simulink model "untitled"  (R2022b)
settings: Solver=FixedStepAuto  StartTime=0.0  StopTime=0.3  FixedStep=1e-7  RelTol=1e-3
undefined symbols (not defined in the file): Ts
libraries: spsMosfetLib x12, simulink x11, spsControlledVoltageSourceLib x1, spsDCVoltageSourceLib x1, spsGroundLib x1, spsPermanentMagnetSynchronousMachineLib x1, spsSVPWMGenerator2LevelLib x1, spsdq0toAlphaBetaZeroLib x1, spspowerguiLib x1
(part 1 of 2)
settings Model: Creator=Javnson  LastModifiedBy=Javnson

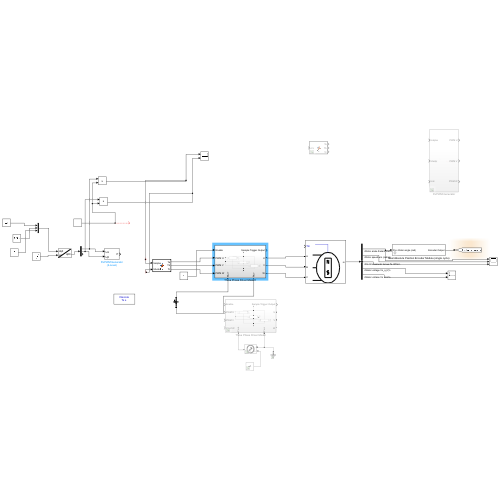
[thumbnail: Simulink's stored preview of the top-level diagram]
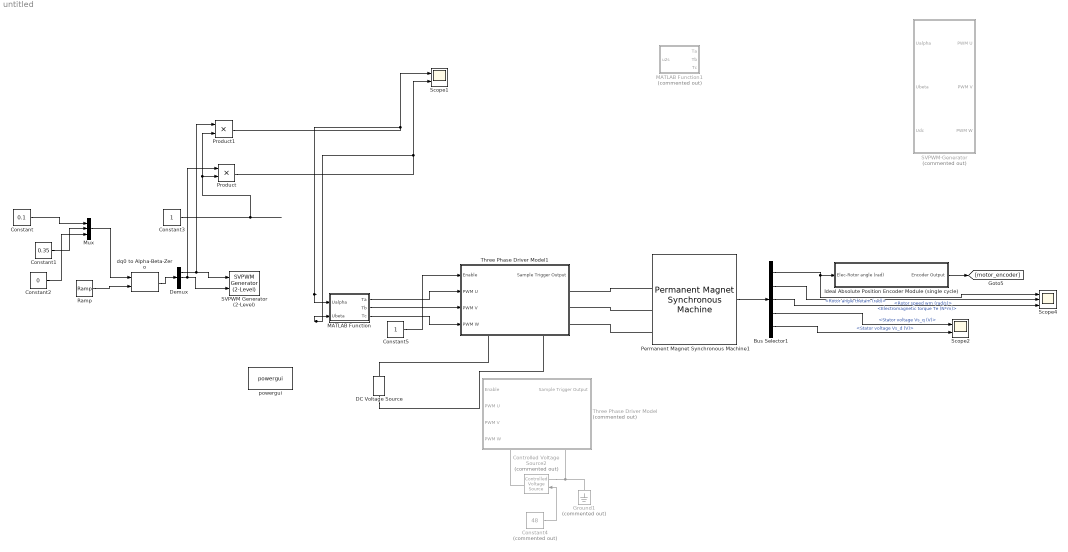
== system untitled ==
  Bus Selector1 : BusSelector  OutputSignals=Rotor angle thetam (rad),Rotor speed wm (rad/s),Electromagnetic torque Te (N*m),Stator voltage Vs_q (V),Stator voltage Vs_d (V)
  Constant : Constant  Value=0.1
  Constant1 : Constant  Value=0.35
  Constant2 : Constant  Value=0
  Constant3 : Constant
  Constant4 : Constant  Commented=on  Value=48
  Constant5 : Constant
  Controlled Voltage Source2 : spsControlledVoltageSourceLib/Controlled Voltage Source  Commented=on  Initialize=on  Source_Type=AC  Amplitude=0  Phase=0  Frequency=0  Measurements=None
  DC Voltage Source : spsDCVoltageSourceLib/DC Voltage Source  Amplitude=48  Measurements=None
  Demux : Demux  Outputs=3
  Ground1 : spsGroundLib/Ground  Commented=on  LConnTagsString=a
  Ideal Absolute Position Encoder Module (single cycle) : Subsystem  mask{ENCODER_BIT=17}
      mask DialogControl DescGroupVar Prompt: Ideal Absolute Position Encoder Module (single cycle)
      mask DialogControl DescTextVar Prompt: Avsolute Encoder transfer a motor mechanical angle (thetam, rad) to Absolute Encoder result. Generally, an absolute encoder has 17-bits or 23-bits resolution results.
      mask DialogControl ParameterGroupVar Prompt: 参数
      mask DialogControl Control2 Prompt: Absolute Encoder Resolution (bits):
  MATLAB Function : MATLAB Function  TreatAsAtomicUnit=on
  MATLAB Function1 : MATLAB Function  Commented=on  TreatAsAtomicUnit=on
  Mux : Mux  Inputs=3
  Permanent Magnet Synchronous Machine1 : spsPermanentMagnetSynchronousMachineLib/Permanent Magnet Synchronous Machine  NbPhases=3  FluxDistribution=Sinusoidal  RotorType=Round  MechanicalLoad=Torque Tm  PresetModel=No  ShowDetailedParameters=on  MeasurementBus=off  Resistance=0.18  Inductance=8.5e-3  dqInductances=[8.5e-3,8.5e-3]  La=0.000835  MachineConstant=Flux linkage established by magnets (V.s)  Flux=0.0714394  VoltageCst=51.8307  TorqueCst=0.42864  Flat=120  Mechanical=[0.000621417 0.000005 4 0]  PolePairs=4  InitialConditions=[0, 0, 0, 0]  InitialConditions5ph=[0 0 0 0 0 0]  RefAngle=Aligned with phase A axis (original Park)  IterativeDiscreteModel=Trapezoidal non iterative  TsBlock=-1  TsPowergui=0
  Product : Product
  Product1 : Product
  Ramp : simulink/Sources/Ramp  slope=40*pi  start=0  InitialOutput=0
  SVPWM Generator (2-Level) : spsSVPWMGenerator2LevelLib/SVPWM Generator (2-Level)  InputType=alpha-beta components  SwitchingPattern=Pattern #2  Fc=10e3  ParUref=[0.8 -30 50]  Ts=0
  SVPWM-Generator : Subsystem  Commented=on
  Scope1 : Scope  NumInputPorts=2
  Scope2 : Scope  NumInputPorts=2
  Scope4 : Scope  NumInputPorts=3
  Three Phase Driver Model : Subsystem  Commented=on
      settings: PortSchema="{\"entries\":[{\"content\":{\"sides\":[{\"content\":{\"connectorIds\":[\"In1\",\"In2\",\"In3\",\"In4\"]},\"type\":\"ConnectorPlacement.EquallySpacedRectSide\",\"uuid\":\"3ffcf095-7a60-4897-81b4-d3692ae6e2ab\"},{\"content\":{\"connectorIds\":[\"Out1\",\"RConn1\",\"RConn2\",\"RConn3\"],\"side\":\"RIGHT\"},\"type\":\"ConnectorPlacement.EquallySpacedRectSide\",\"uuid\":\"6e5cf4cf-b1b9-48ac-a692-0a8874277a23\"},{\"content\":{\"connectorIds\":[],\"side\":\"TOP\"},\"type\":\"ConnectorPlacement.EquallySpacedRectSide\",\"uuid\":\"9aa765f5-1b2f-406c-a04a-fab38ac2c4f7\"},{\"content\":{\"connectorIds\":[\"RConn4\",\"RConn5\"],\"side\":\"BOTTOM\"},\"type\":\"ConnectorPlacement.EquallySpacedRectSide\",\"uuid\":\"ff3856e6-d154-4ba2-8db0-f3c94a45cad8\"}]},\"type\":\"ConnectorPlacement.EquallySpacedConnector\",\"uuid\":\"490a993e-7d06-4faf-ab4a-bafd9b6172f2\"}],\"packageUris\":[\"http://schema.mathworks.com/mf0/Connector/R2020b\"],\"version\":\"1.0\"}"
  Three Phase Driver Model1 : Subsystem
      settings: PortSchema="{\"entries\":[{\"content\":{\"sides\":[{\"content\":{\"connectorIds\":[\"In1\",\"In2\",\"In3\",\"In4\"]},\"type\":\"ConnectorPlacement.EquallySpacedRectSide\",\"uuid\":\"3ffcf095-7a60-4897-81b4-d3692ae6e2ab\"},{\"content\":{\"connectorIds\":[\"Out1\",\"RConn1\",\"RConn2\",\"RConn3\"],\"side\":\"RIGHT\"},\"type\":\"ConnectorPlacement.EquallySpacedRectSide\",\"uuid\":\"6e5cf4cf-b1b9-48ac-a692-0a8874277a23\"},{\"content\":{\"connectorIds\":[],\"side\":\"TOP\"},\"type\":\"ConnectorPlacement.EquallySpacedRectSide\",\"uuid\":\"9aa765f5-1b2f-406c-a04a-fab38ac2c4f7\"},{\"content\":{\"connectorIds\":[\"RConn4\",\"RConn5\"],\"side\":\"BOTTOM\"},\"type\":\"ConnectorPlacement.EquallySpacedRectSide\",\"uuid\":\"ff3856e6-d154-4ba2-8db0-f3c94a45cad8\"}]},\"type\":\"ConnectorPlacement.EquallySpacedConnector\",\"uuid\":\"490a993e-7d06-4faf-ab4a-bafd9b6172f2\"}],\"packageUris\":[\"http://schema.mathworks.com/mf0/Connector/R2020b\"],\"version\":\"1.0\"}"
  dq0 to Alpha-Beta-Zero : spsdq0toAlphaBetaZeroLib/dq0 to Alpha-Beta-Zero  Alignment=Aligned with phase A axis
  powergui : spspowerguiLib/powergui  Priority=1  SimulationMode=Discrete  SampleTime=Ts  frequency=60  Iterations=50  frequencyindice=0  Pbase=100e6  ErrMax=1e-4  UnitsV=kV  UnitsW=MW  buscounter=0  FunctionMessages=off  echomessages=off  EnableUseOfTLC=off  CurrentSourceSwitches=off  DisableSnubberDevices=off  DisableRonSwitches=off  DisableVfSwitches=off  DisplayEquations=off  AutomaticDiscreteSolvers=off  SolverType=Tustin/Backward Euler (TBE)  Interpol=off  ExternalGateDelay=off  methode=off  Ts=100  x0status=blocks  SPID=on  SwTol=0  HookPort=off  NonlinearTolerance=1e-4  nMaxIteration=100  ContinueOnMaxIteration=off  RestoreLinks=warning  ResistiveCurrentMeasurement=off  Frange=[0:2:500]  Ylog=off  Xlog=on  ShowGrid=off  save=off  variable=ZData  structure=0  ZoomFFT=off  StartTime=0.0  cycles=1  DisplayStyle=1  fundamental=60  FreqAxis=off  MaxFrequency=1000  frequencyindicesteady=1  RmsSteady=1  display=off
  wires:
  Demux/1 -> Product1/1, SVPWM Generator (2-Level)/1
  Demux/2 -> Product/1, SVPWM Generator (2-Level)/2
  dq0 to Alpha-Beta-Zero/1 -> Demux/1
  Ramp/1 -> dq0 to Alpha-Beta-Zero/2
  Mux/1 -> dq0 to Alpha-Beta-Zero/1
  Constant/1 -> Mux/1
  Constant1/1 -> Mux/2
  Constant2/1 -> Mux/3
  Bus Selector1/2 -> Scope4/2  "<Rotor speed wm (rad/s)>"
  Bus Selector1/4 -> Scope2/1  "<Stator voltage Vs_q (V)>"
  Bus Selector1/5 -> Scope2/2  "<Stator voltage Vs_d (V)>"
  Ideal Absolute Position Encoder Module (single cycle)/1(Encoder Output) -> [motor_encoder]
  Permanent Magnet Synchronous Machine1/1 -> Bus Selector1/1
  Bus Selector1/1 -> Scope4/1, Ideal Absolute Position Encoder Module (single cycle)/1(Elec-Rotor angle (rad))  "<Rotor angle thetam (rad)>"
  Bus Selector1/3 -> Scope4/3  "<Electromagnetic torque Te (N*m)>"
  Constant4/1 -> Controlled Voltage Source2/1
  Product/1 -> MATLAB Function/2(Ubeta), Scope1/2
  Constant3/1 -> Product/2, Product1/2
  MATLAB Function/1(Ta) -> Three Phase Driver Model1/2(PWM U)
  MATLAB Function/2(Tb) -> Three Phase Driver Model1/3(PWM V)
  MATLAB Function/3(Tc) -> Three Phase Driver Model1/4(PWM W)
  Constant5/1 -> Three Phase Driver Model1/1(Enable)
  Product1/1 -> Scope1/1, MATLAB Function/1(Ualpha)
  connections:
  Permanent Magnet Synchronous Machine1/LConn1 -- Three Phase Driver Model1/RConn1
  Permanent Magnet Synchronous Machine1/LConn2 -- Three Phase Driver Model1/RConn2
  Permanent Magnet Synchronous Machine1/LConn3 -- Three Phase Driver Model1/RConn3
  DC Voltage Source/RConn1 -- Three Phase Driver Model1/RConn4
  DC Voltage Source/LConn1 -- Three Phase Driver Model1/RConn5
  Ground1/LConn1 -- Controlled Voltage Source2/LConn1 -- Three Phase Driver Model/RConn5
  Controlled Voltage Source2/RConn1 -- Three Phase Driver Model/RConn4

== system untitled/Ideal Absolute Position Encoder Module (single cycle) ==
  Elec-Rotor angle (rad) : Inport
  Data Type Conversion : DataTypeConversion  OutDataTypeStr=uint32  SaturateOnIntegerOverflow=off  RndMeth=Floor
  Gain : Gain  Gain=1/2/pi
  Type Conversion : Gain  Gain=2^ENCODER_BIT
  Encoder Output : Outport
  wires:
  Gain/1 -> Type Conversion/1
  Type Conversion/1 -> Data Type Conversion/1
  Data Type Conversion/1 -> Encoder Output/1
  Elec-Rotor angle (rad)/1 -> Gain/1

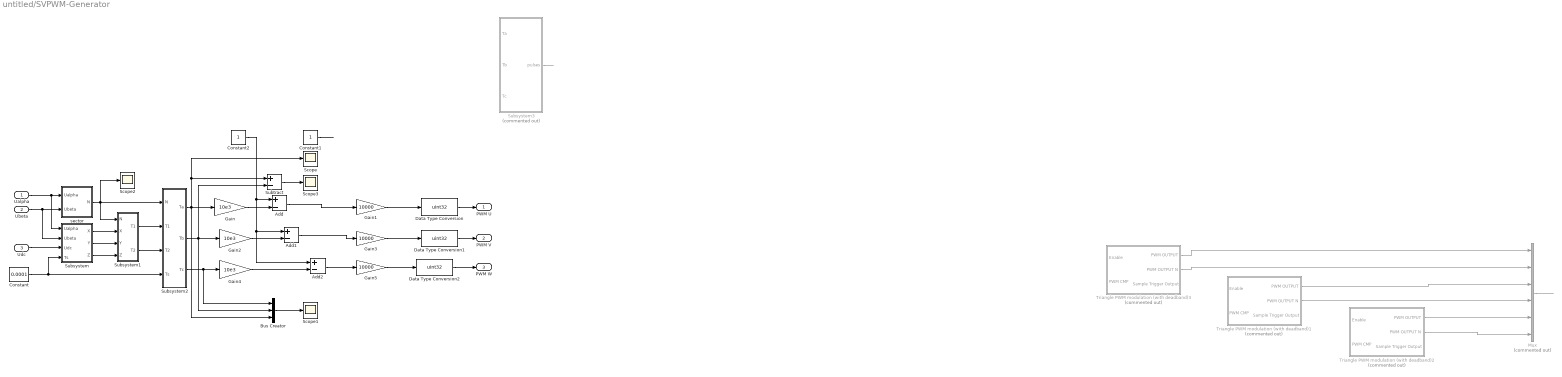
== system untitled/SVPWM-Generator ==
  Ualpha : Inport
  Ubeta : Inport  Port=2
  Udc : Inport  Port=3
  Add : Sum  Inputs=+-
  Add1 : Sum  Inputs=+-
  Add2 : Sum  Inputs=+-
  Bus Creator : BusCreator  Inputs=3
  Constant : Constant  Value=0.0001
  Constant1 : Constant
  Constant2 : Constant
  Data Type Conversion : DataTypeConversion  OutDataTypeStr=uint32  SaturateOnIntegerOverflow=off  RndMeth=Floor
  Data Type Conversion1 : DataTypeConversion  OutDataTypeStr=uint32  SaturateOnIntegerOverflow=off  RndMeth=Floor
  Data Type Conversion2 : DataTypeConversion  OutDataTypeStr=uint32  SaturateOnIntegerOverflow=off  RndMeth=Floor
  Gain : Gain  Gain=10e3
  Gain1 : Gain  Gain=10000
  Gain2 : Gain  Gain=10e3
  Gain3 : Gain  Gain=10000
  Gain4 : Gain  Gain=10e3
  Gain5 : Gain  Gain=10000
  Mux : Mux  Commented=on  Inputs=6
  Scope{,1..3} (4 alike) : Scope
  Subsystem : Subsystem
  Subsystem1 : Subsystem
  Subsystem2 : Subsystem
  Subsystem3 : Subsystem  Commented=on
  Subtract : Sum  Inputs=+-
  Triangle PWM modulation (with deadband)1 : Subsystem  Commented=on  mask{fswitch=10e3, CMP_MAX=10000, Deadband_Upper=0, Deadband_Lower=0, Parameter4=0}
      mask prompts: Parameter4 "Deadband Time: (μs)"
      mask Callback Deadband_Upper: %dead_cmp_param = get_param('DEADBAND_CMP','Value');
      mask DialogControl DescGroupVar Prompt: PWM Modulator
      mask DialogControl DescTextVar Prompt: PWM Modulator. Input PWM compare register value, output ADC trigger signal, PWM output and negtive PWM output.
      mask DialogControl ParameterGroupVar Prompt: 参数
      mask DialogControl Control2 Prompt: PWM Frequency (Hz) :
      mask DialogControl Control4 Prompt: Full Scale PWM Compare value:
      mask DialogControl Control5 Prompt: (whole period is 2 * CMP_MAX ticks)
      mask DialogControl Control3 Prompt: Deadband Range Set (CMP Value):
      mask DialogControl Control6 Prompt: Single side deadband time: DEADBAND_CMP/2/CMP_MAX/fswitch
  Triangle PWM modulation (with deadband)2 : Subsystem  Commented=on  mask{fswitch=10e3, CMP_MAX=10000, Deadband_Upper=0, Deadband_Lower=0, Parameter4=0}
      mask prompts: Parameter4 "Deadband Time: (μs)"
      mask Callback Deadband_Upper: %dead_cmp_param = get_param('DEADBAND_CMP','Value');
      mask DialogControl DescGroupVar Prompt: PWM Modulator
      mask DialogControl DescTextVar Prompt: PWM Modulator. Input PWM compare register value, output ADC trigger signal, PWM output and negtive PWM output.
      mask DialogControl ParameterGroupVar Prompt: 参数
      mask DialogControl Control2 Prompt: PWM Frequency (Hz) :
      mask DialogControl Control4 Prompt: Full Scale PWM Compare value:
      mask DialogControl Control5 Prompt: (whole period is 2 * CMP_MAX ticks)
      mask DialogControl Control3 Prompt: Deadband Range Set (CMP Value):
      mask DialogControl Control6 Prompt: Single side deadband time: DEADBAND_CMP/2/CMP_MAX/fswitch
  Triangle PWM modulation (with deadband)3 : Subsystem  Commented=on  mask{fswitch=10e3, CMP_MAX=10000, Deadband_Upper=0, Deadband_Lower=0, Parameter4=0}
      mask prompts: Parameter4 "Deadband Time: (μs)"
      mask Callback Deadband_Upper: %dead_cmp_param = get_param('DEADBAND_CMP','Value');
      mask DialogControl DescGroupVar Prompt: PWM Modulator
      mask DialogControl DescTextVar Prompt: PWM Modulator. Input PWM compare register value, output ADC trigger signal, PWM output and negtive PWM output.
      mask DialogControl ParameterGroupVar Prompt: 参数
      mask DialogControl Control2 Prompt: PWM Frequency (Hz) :
      mask DialogControl Control4 Prompt: Full Scale PWM Compare value:
      mask DialogControl Control5 Prompt: (whole period is 2 * CMP_MAX ticks)
      mask DialogControl Control3 Prompt: Deadband Range Set (CMP Value):
      mask DialogControl Control6 Prompt: Single side deadband time: DEADBAND_CMP/2/CMP_MAX/fswitch
  sector : Subsystem
  PWM U : Outport
  PWM V : Outport  Port=2
  PWM W : Outport  Port=3
  wires:
  sector/1(N) -> Scope2/1, Subsystem2/1(N), Subsystem1/1(N)
  Subsystem2/3(Tc) -> Gain4/1, Bus Creator/1
  Subsystem1/1(T1) -> Subsystem2/2(T1)
  Subsystem1/2(T2) -> Subsystem2/3(T2)
  Subsystem/1(X) -> Subsystem1/2(X)
  Subsystem3/1(pulses) -> ?
  Ubeta/1 -> Subsystem/2(Ubeta), sector/2(Ubeta)
  Constant/1 -> Subsystem2/4(Ts), Subsystem/4(Ts)
  Subsystem/2(Y) -> Subsystem1/3(Y)
  Subsystem/3(Z) -> Subsystem1/4(Z)
  Ualpha/1 -> Subsystem/1(Ualpha), sector/1(Ualpha)
  Subsystem2/1(Ta) -> Gain/1, Bus Creator/3, Subtract/1, Scope/1
  Udc/1 -> Subsystem/3(Udc)
  Bus Creator/1 -> Scope1/1
  Subtract/1 -> Scope3/1
  Gain1/1 -> Data Type Conversion/1
  Gain5/1 -> Data Type Conversion2/1
  Gain3/1 -> Data Type Conversion1/1
  Subsystem2/2(Tb) -> Gain2/1, Subtract/2, Bus Creator/2
  Constant1/1 -> ?
  Add/1 -> Gain1/1
  Gain/1 -> Add/2
  Add1/1 -> Gain3/1
  Gain2/1 -> Add1/2
  Add2/1 -> Gain5/1
  Gain4/1 -> Add2/2
  Constant2/1 -> Add2/1, Add1/1, Add/1
  Triangle PWM modulation (with deadband)2/2(PWM OUTPUT N) -> Mux/6
  ? -> Triangle PWM modulation (with deadband)1/1(Enable), Triangle PWM modulation (with deadband)2/1(Enable)
  ? -> Triangle PWM modulation (with deadband)3/1(Enable)
  Triangle PWM modulation (with deadband)1/1(PWM OUTPUT) -> Mux/3
  Mux/1 -> ?
  Triangle PWM modulation (with deadband)2/1(PWM OUTPUT) -> Mux/5
  Triangle PWM modulation (with deadband)3/2(PWM OUTPUT N) -> Mux/2
  ? -> Triangle PWM modulation (with deadband)1/2(PWM CMP)
  Triangle PWM modulation (with deadband)1/2(PWM OUTPUT N) -> Mux/4
  ? -> Triangle PWM modulation (with deadband)2/2(PWM CMP)
  Triangle PWM modulation (with deadband)3/1(PWM OUTPUT) -> Mux/1
  ? -> Triangle PWM modulation (with deadband)3/2(PWM CMP)
  Data Type Conversion/1 -> PWM U/1
  Data Type Conversion1/1 -> PWM V/1
  Data Type Conversion2/1 -> PWM W/1

== system untitled/Three Phase Driver Model ==
  Enable : Inport
  PWM U : Inport  Port=2
  PWM V : Inport  Port=3
  PWM W : Inport  Port=4
  Single Phase Full Bridge : Subsystem
      settings: PortSchema="{\"entries\":[{\"content\":{\"sides\":[{\"content\":{\"connectorIds\":[\"In1\",\"In2\"]},\"type\":\"ConnectorPlacement.EquallySpacedRectSide\",\"uuid\":\"20beeabc-b0ca-4337-b227-c7f02abd15d8\"},{\"content\":{\"connectorIds\":[\"Out1\",\"RConn1\"],\"side\":\"RIGHT\"},\"type\":\"ConnectorPlacement.EquallySpacedRectSide\",\"uuid\":\"a7923383-ac55-4621-ad1d-4d067c1fb84d\"},{\"content\":{\"connectorIds\":[\"LConn1\"],\"side\":\"TOP\"},\"type\":\"ConnectorPlacement.EquallySpacedRectSide\",\"uuid\":\"661bf0ae-1c96-4de8-96aa-28c06a0a56db\"},{\"content\":{\"connectorIds\":[\"RConn2\"],\"side\":\"BOTTOM\"},\"type\":\"ConnectorPlacement.EquallySpacedRectSide\",\"uuid\":\"fc2f6321-5787-4e1a-b5a2-65ed34db36b5\"}]},\"type\":\"ConnectorPlacement.EquallySpacedConnector\",\"uuid\":\"e2219b16-0a50-43ef-8183-c55a35d5a2a0\"}],\"packageUris\":[\"http://schema.mathworks.com/mf0/Connector/R2020b\"],\"version\":\"1.0\"}"
  Single Phase Full Bridge1 : Subsystem
      settings: PortSchema="{\"entries\":[{\"content\":{\"sides\":[{\"content\":{\"connectorIds\":[\"In1\",\"In2\"]},\"type\":\"ConnectorPlacement.EquallySpacedRectSide\",\"uuid\":\"20beeabc-b0ca-4337-b227-c7f02abd15d8\"},{\"content\":{\"connectorIds\":[\"Out1\",\"RConn1\"],\"side\":\"RIGHT\"},\"type\":\"ConnectorPlacement.EquallySpacedRectSide\",\"uuid\":\"a7923383-ac55-4621-ad1d-4d067c1fb84d\"},{\"content\":{\"connectorIds\":[\"LConn1\"],\"side\":\"TOP\"},\"type\":\"ConnectorPlacement.EquallySpacedRectSide\",\"uuid\":\"661bf0ae-1c96-4de8-96aa-28c06a0a56db\"},{\"content\":{\"connectorIds\":[\"RConn2\"],\"side\":\"BOTTOM\"},\"type\":\"ConnectorPlacement.EquallySpacedRectSide\",\"uuid\":\"fc2f6321-5787-4e1a-b5a2-65ed34db36b5\"}]},\"type\":\"ConnectorPlacement.EquallySpacedConnector\",\"uuid\":\"e2219b16-0a50-43ef-8183-c55a35d5a2a0\"}],\"packageUris\":[\"http://schema.mathworks.com/mf0/Connector/R2020b\"],\"version\":\"1.0\"}"
  Single Phase Full Bridge2 : Subsystem
      settings: PortSchema="{\"entries\":[{\"content\":{\"sides\":[{\"content\":{\"connectorIds\":[\"In1\",\"In2\"]},\"type\":\"ConnectorPlacement.EquallySpacedRectSide\",\"uuid\":\"20beeabc-b0ca-4337-b227-c7f02abd15d8\"},{\"content\":{\"connectorIds\":[\"Out1\",\"RConn1\"],\"side\":\"RIGHT\"},\"type\":\"ConnectorPlacement.EquallySpacedRectSide\",\"uuid\":\"a7923383-ac55-4621-ad1d-4d067c1fb84d\"},{\"content\":{\"connectorIds\":[\"LConn1\"],\"side\":\"TOP\"},\"type\":\"ConnectorPlacement.EquallySpacedRectSide\",\"uuid\":\"661bf0ae-1c96-4de8-96aa-28c06a0a56db\"},{\"content\":{\"connectorIds\":[\"RConn2\"],\"side\":\"BOTTOM\"},\"type\":\"ConnectorPlacement.EquallySpacedRectSide\",\"uuid\":\"fc2f6321-5787-4e1a-b5a2-65ed34db36b5\"}]},\"type\":\"ConnectorPlacement.EquallySpacedConnector\",\"uuid\":\"e2219b16-0a50-43ef-8183-c55a35d5a2a0\"}],\"packageUris\":[\"http://schema.mathworks.com/mf0/Connector/R2020b\"],\"version\":\"1.0\"}"
  Terminator : Terminator
  Terminator1 : Terminator
  U : PMIOPort  Side=Right
  V : PMIOPort  Port=2  Side=Right
  W : PMIOPort  Port=3  Side=Right
  Pwr+ : PMIOPort  Port=4  Side=Right
  Pwr- : PMIOPort  Port=5  Side=Right
  Sample Trigger Output : Outport
  wires:
  PWM W/1 -> Single Phase Full Bridge2/2(PWM CMP)
  Single Phase Full Bridge2/1(Sample Trigger Output) -> Terminator1/1
  Enable/1 -> Single Phase Full Bridge/1(Enable), Single Phase Full Bridge1/1(Enable), Single Phase Full Bridge2/1(Enable)
  Single Phase Full Bridge1/1(Sample Trigger Output) -> Terminator/1
  Single Phase Full Bridge/1(Sample Trigger Output) -> Sample Trigger Output/1
  PWM U/1 -> Single Phase Full Bridge/2(PWM CMP)
  PWM V/1 -> Single Phase Full Bridge1/2(PWM CMP)
  connections:
  Single Phase Full Bridge2/LConn1 -- Pwr+/RConn1 -- Single Phase Full Bridge1/LConn1 -- Single Phase Full Bridge/LConn1
  Single Phase Full Bridge2/RConn2 -- Pwr-/RConn1 -- Single Phase Full Bridge/RConn2 -- Single Phase Full Bridge1/RConn2
  Single Phase Full Bridge1/RConn1 -- V/RConn1
  Single Phase Full Bridge2/RConn1 -- W/RConn1
  Single Phase Full Bridge/RConn1 -- U/RConn1

== system untitled/Three Phase Driver Model1 ==
  Enable : Inport
  PWM U : Inport  Port=2
  PWM V : Inport  Port=3
  PWM W : Inport  Port=4
  Single Phase Full Bridge : Subsystem
      settings: PortSchema="{\"entries\":[{\"content\":{\"sides\":[{\"content\":{\"connectorIds\":[\"In1\",\"In2\"]},\"type\":\"ConnectorPlacement.EquallySpacedRectSide\",\"uuid\":\"20beeabc-b0ca-4337-b227-c7f02abd15d8\"},{\"content\":{\"connectorIds\":[\"Out1\",\"RConn1\"],\"side\":\"RIGHT\"},\"type\":\"ConnectorPlacement.EquallySpacedRectSide\",\"uuid\":\"a7923383-ac55-4621-ad1d-4d067c1fb84d\"},{\"content\":{\"connectorIds\":[\"LConn1\"],\"side\":\"TOP\"},\"type\":\"ConnectorPlacement.EquallySpacedRectSide\",\"uuid\":\"661bf0ae-1c96-4de8-96aa-28c06a0a56db\"},{\"content\":{\"connectorIds\":[\"RConn2\"],\"side\":\"BOTTOM\"},\"type\":\"ConnectorPlacement.EquallySpacedRectSide\",\"uuid\":\"fc2f6321-5787-4e1a-b5a2-65ed34db36b5\"}]},\"type\":\"ConnectorPlacement.EquallySpacedConnector\",\"uuid\":\"e2219b16-0a50-43ef-8183-c55a35d5a2a0\"}],\"packageUris\":[\"http://schema.mathworks.com/mf0/Connector/R2020b\"],\"version\":\"1.0\"}"
  Single Phase Full Bridge1 : Subsystem
      settings: PortSchema="{\"entries\":[{\"content\":{\"sides\":[{\"content\":{\"connectorIds\":[\"In1\",\"In2\"]},\"type\":\"ConnectorPlacement.EquallySpacedRectSide\",\"uuid\":\"20beeabc-b0ca-4337-b227-c7f02abd15d8\"},{\"content\":{\"connectorIds\":[\"Out1\",\"RConn1\"],\"side\":\"RIGHT\"},\"type\":\"ConnectorPlacement.EquallySpacedRectSide\",\"uuid\":\"a7923383-ac55-4621-ad1d-4d067c1fb84d\"},{\"content\":{\"connectorIds\":[\"LConn1\"],\"side\":\"TOP\"},\"type\":\"ConnectorPlacement.EquallySpacedRectSide\",\"uuid\":\"661bf0ae-1c96-4de8-96aa-28c06a0a56db\"},{\"content\":{\"connectorIds\":[\"RConn2\"],\"side\":\"BOTTOM\"},\"type\":\"ConnectorPlacement.EquallySpacedRectSide\",\"uuid\":\"fc2f6321-5787-4e1a-b5a2-65ed34db36b5\"}]},\"type\":\"ConnectorPlacement.EquallySpacedConnector\",\"uuid\":\"e2219b16-0a50-43ef-8183-c55a35d5a2a0\"}],\"packageUris\":[\"http://schema.mathworks.com/mf0/Connector/R2020b\"],\"version\":\"1.0\"}"
  Single Phase Full Bridge2 : Subsystem
      settings: PortSchema="{\"entries\":[{\"content\":{\"sides\":[{\"content\":{\"connectorIds\":[\"In1\",\"In2\"]},\"type\":\"ConnectorPlacement.EquallySpacedRectSide\",\"uuid\":\"20beeabc-b0ca-4337-b227-c7f02abd15d8\"},{\"content\":{\"connectorIds\":[\"Out1\",\"RConn1\"],\"side\":\"RIGHT\"},\"type\":\"ConnectorPlacement.EquallySpacedRectSide\",\"uuid\":\"a7923383-ac55-4621-ad1d-4d067c1fb84d\"},{\"content\":{\"connectorIds\":[\"LConn1\"],\"side\":\"TOP\"},\"type\":\"ConnectorPlacement.EquallySpacedRectSide\",\"uuid\":\"661bf0ae-1c96-4de8-96aa-28c06a0a56db\"},{\"content\":{\"connectorIds\":[\"RConn2\"],\"side\":\"BOTTOM\"},\"type\":\"ConnectorPlacement.EquallySpacedRectSide\",\"uuid\":\"fc2f6321-5787-4e1a-b5a2-65ed34db36b5\"}]},\"type\":\"ConnectorPlacement.EquallySpacedConnector\",\"uuid\":\"e2219b16-0a50-43ef-8183-c55a35d5a2a0\"}],\"packageUris\":[\"http://schema.mathworks.com/mf0/Connector/R2020b\"],\"version\":\"1.0\"}"
  Terminator : Terminator
  Terminator1 : Terminator
  U : PMIOPort  Side=Right
  V : PMIOPort  Port=2  Side=Right
  W : PMIOPort  Port=3  Side=Right
  Pwr+ : PMIOPort  Port=4  Side=Right
  Pwr- : PMIOPort  Port=5  Side=Right
  Sample Trigger Output : Outport
  wires:
  PWM W/1 -> Single Phase Full Bridge2/2(PWM CMP)
  Single Phase Full Bridge2/1(Sample Trigger Output) -> Terminator1/1
  Enable/1 -> Single Phase Full Bridge/1(Enable), Single Phase Full Bridge1/1(Enable), Single Phase Full Bridge2/1(Enable)
  Single Phase Full Bridge1/1(Sample Trigger Output) -> Terminator/1
  Single Phase Full Bridge/1(Sample Trigger Output) -> Sample Trigger Output/1
  PWM U/1 -> Single Phase Full Bridge/2(PWM CMP)
  PWM V/1 -> Single Phase Full Bridge1/2(PWM CMP)
  connections:
  Single Phase Full Bridge2/LConn1 -- Pwr+/RConn1 -- Single Phase Full Bridge1/LConn1 -- Single Phase Full Bridge/LConn1
  Single Phase Full Bridge2/RConn2 -- Pwr-/RConn1 -- Single Phase Full Bridge/RConn2 -- Single Phase Full Bridge1/RConn2
  Single Phase Full Bridge1/RConn1 -- V/RConn1
  Single Phase Full Bridge2/RConn1 -- W/RConn1
  Single Phase Full Bridge/RConn1 -- U/RConn1

== system untitled/SVPWM-Generator/Subsystem ==
  Ualpha : Inport
  Ubeta : Inport  Port=2
  Udc : Inport  Port=3
  Ts : Inport  Port=4
  Add : Sum
  Constant : Constant  Value=1.5
  Constant1 : Constant  Value=0.866
  Constant2 : Constant  Value=1.732
  Math Function : Math  Operator=reciprocal
  Product{,1..6} (7 alike) : Product
  Subtract : Sum  Inputs=+-
  X : Outport
  Y : Outport  Port=2
  Z : Outport  Port=3
  wires:
  Product1/1 -> Product4/2, Product5/2, Product6/2
  Ts/1 -> Product1/2
  Product6/1 -> Z/1
  Add/1 -> Product5/1
  Ualpha/1 -> Product/2
  Math Function/1 -> Product1/1
  Product2/1 -> Subtract/1, Add/2
  Product4/1 -> X/1
  Product3/1 -> Product4/1
  Constant/1 -> Product/1
  Constant1/1 -> Product2/1
  Ubeta/1 -> Product3/1, Product2/2
  Product5/1 -> Y/1
  Product/1 -> Add/1, Subtract/2
  Constant2/1 -> Product3/2
  Udc/1 -> Math Function/1
  Subtract/1 -> Product6/1

== system untitled/SVPWM-Generator/Subsystem1 ==
  N : Inport
  X : Inport  Port=2
  Y : Inport  Port=3
  Z : Inport  Port=4
  Gain : Gain  Gain=-1
  Gain1 : Gain  Gain=-1
  Gain2 : Gain  Gain=-1
  Multiport Switch : MultiPortSwitch  Inputs=6  SaturateOnIntegerOverflow=off  InputSameDT=off
  Multiport Switch1 : MultiPortSwitch  Inputs=6  SaturateOnIntegerOverflow=off  InputSameDT=off
  T1 : Outport
  T2 : Outport  Port=2
  wires:
  Multiport Switch1/1 -> T2/1
  X/1 -> Multiport Switch1/4, Multiport Switch/6, Gain/1
  Y/1 -> Gain1/1, Multiport Switch/3, Multiport Switch1/2
  Z/1 -> Gain2/1, Multiport Switch/2, Multiport Switch1/5
  Gain/1 -> Multiport Switch1/3, Multiport Switch/5
  Gain2/1 -> Multiport Switch/4, Multiport Switch1/7
  N/1 -> Multiport Switch1/1, Multiport Switch/1
  Gain1/1 -> Multiport Switch1/6, Multiport Switch/7
  Multiport Switch/1 -> T1/1

== system untitled/SVPWM-Generator/Subsystem2 ==
  N : Inport
  T1 : Inport  Port=2  Interpolate=off
  T2 : Inport  Port=3
  Ts : Inport  Port=4
  Add : Sum
  Add1 : Sum
  Constant : Constant  Value=0.25
  Constant1 : Constant  Value=0.5
  Constant2 : Constant  Value=0.5
  Multiport Switch : MultiPortSwitch  Inputs=6  SaturateOnIntegerOverflow=off  InputSameDT=off
  Multiport Switch1 : MultiPortSwitch  Inputs=6  SaturateOnIntegerOverflow=off  InputSameDT=off
  Multiport Switch2 : MultiPortSwitch  Inputs=6  SaturateOnIntegerOverflow=off  InputSameDT=off
  Product : Product
  Product1 : Product
  Product2 : Product
  Subtract : Sum  Inputs=--+
  Ta : Outport
  Tb : Outport  Port=2
  Tc : Outport  Port=3
  wires:
  Subtract/1 -> Product/1
  Product1/1 -> Add1/1
  T2/1 -> Product1/1, Subtract/2
  Product/1 -> Add/2, Multiport Switch2/5, Multiport Switch2/7, Multiport Switch/4, Multiport Switch/3, Multiport Switch1/2, Multiport Switch1/6
  Multiport Switch2/1 -> Tc/1
  Add1/1 -> Multiport Switch2/4, Multiport Switch2/2, Multiport Switch1/7, Multiport Switch1/3, Multiport Switch/6, Multiport Switch/5
  N/1 -> Multiport Switch2/1, Multiport Switch1/1, Multiport Switch/1
  Multiport Switch/1 -> Ta/1
  Constant/1 -> Product/2
  Constant2/1 -> Product2/2
  Add/1 -> Add1/2, Multiport Switch1/5, Multiport Switch/7, Multiport Switch/2, Multiport Switch1/4, Multiport Switch2/6, Multiport Switch2/3
  Multiport Switch1/1 -> Tb/1
  Product2/1 -> Add/1
  Constant1/1 -> Product1/2
  T1/1 -> Product2/1, Subtract/1
  Ts/1 -> Subtract/3

== system untitled/SVPWM-Generator/Subsystem3 ==
  Ta : Inport
  Tb : Inport  Port=2
  Tc : Inport  Port=3
  Bus Creator : BusCreator  Inputs=2
  Data Type Conversion : DataTypeConversion  OutDataTypeStr=boolean  SaturateOnIntegerOverflow=off  RndMeth=Floor  LockScale=on
  Data Type Conversion1 : DataTypeConversion  OutDataTypeStr=boolean  SaturateOnIntegerOverflow=off  RndMeth=Floor  LockScale=on
  Data Type Conversion2 : DataTypeConversion  OutDataTypeStr=boolean  SaturateOnIntegerOverflow=off  RndMeth=Floor  LockScale=on
  Logical Operator : Logic  Operator=NOT  AllPortsSameDT=off  OutDataTypeStr=boolean
  Logical Operator1 : Logic  Operator=NOT  AllPortsSameDT=off  OutDataTypeStr=boolean
  Logical Operator2 : Logic  Operator=NOT  AllPortsSameDT=off  OutDataTypeStr=boolean
  Mux : Mux  Inputs=6
  Relay : Relay
  Relay1 : Relay
  Relay2 : Relay
  Repeating Sequence : simulink/Sources/Repeating Sequence  rep_seq_t=[0 0.0001 0.0002]  rep_seq_y=[0 0.0001 0]
  Scope : Scope
  Subtract : Sum  Inputs=-+
  Subtract1 : Sum  Inputs=-+
  Subtract2 : Sum  Inputs=-+
  pulses : Outport
  wires:
  Data Type Conversion2/1 -> Mux/5
  Subtract1/1 -> Relay1/1
  Mux/1 -> pulses/1
  Data Type Conversion1/1 -> Mux/3
  Logical Operator2/1 -> Mux/6
  Relay/1 -> Logical Operator/1, Data Type Conversion/1
  Relay2/1 -> Logical Operator2/1, Data Type Conversion2/1
  Logical Operator/1 -> Bus Creator/2, Mux/2
  Relay1/1 -> Logical Operator1/1, Data Type Conversion1/1
  Repeating Sequence/1 -> Subtract/2, Subtract1/2, Subtract2/2
  Data Type Conversion/1 -> Bus Creator/1, Mux/1
  Logical Operator1/1 -> Mux/4
  Ta/1 -> Subtract/1
  Subtract2/1 -> Relay2/1
  Tb/1 -> Subtract1/1
  Subtract/1 -> Relay/1
  Tc/1 -> Subtract2/1
  Bus Creator/1 -> Scope/1

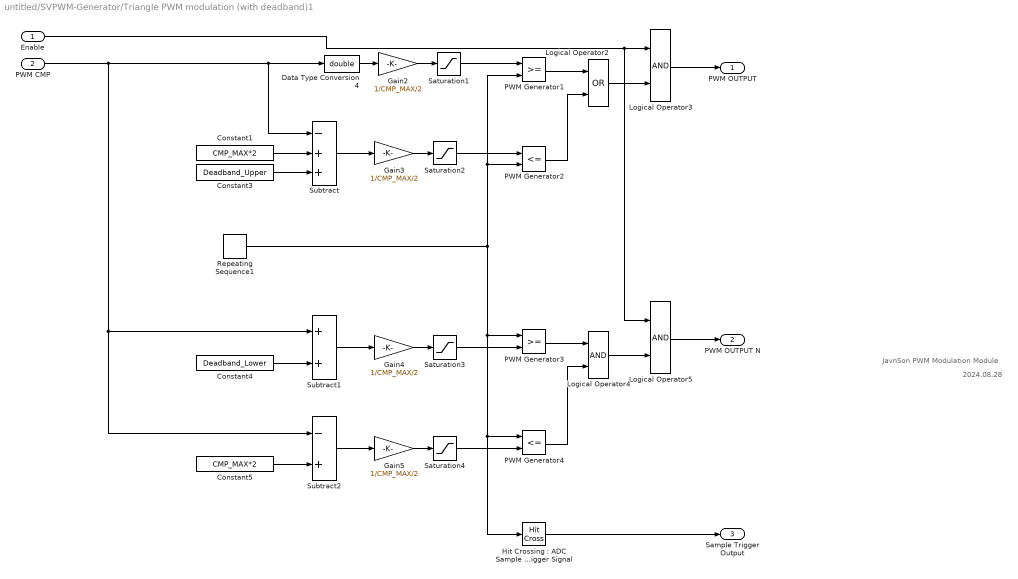
== system untitled/SVPWM-Generator/Triangle PWM modulation (with deadband)1 ==
  note: 2024.08.28
  note: JavnSon PWM Modulation Module
  Enable : Inport
  PWM CMP : Inport  Port=2
  Constant1 : Constant  Value=CMP_MAX*2
  Constant3 : Constant  Value=Deadband_Upper
  Constant4 : Constant  Value=Deadband_Lower
  Constant5 : Constant  Value=CMP_MAX*2
  Data Type Conversion4 : DataTypeConversion  OutDataTypeStr=double  SaturateOnIntegerOverflow=off  RndMeth=Floor
  Gain{2..5} (4 alike) : Gain  Gain=1/CMP_MAX/2
  Hit Crossing：ADC Sample Trigger Signal : HitCross  HitCrossingOffset=0.5  HitCrossingDirection=rising
  Logical Operator2 : Logic  Operator=OR  AllPortsSameDT=off  OutDataTypeStr=boolean
  Logical Operator3 : Logic  AllPortsSameDT=off  OutDataTypeStr=boolean
  Logical Operator4 : Logic  AllPortsSameDT=off  OutDataTypeStr=boolean
  Logical Operator5 : Logic  AllPortsSameDT=off  OutDataTypeStr=boolean
  PWM Generator1 : RelationalOperator  OutDataTypeStr=boolean  InputSameDT=off
  PWM Generator2 : RelationalOperator  Operator=<=  OutDataTypeStr=boolean  InputSameDT=off
  PWM Generator3 : RelationalOperator  OutDataTypeStr=boolean  InputSameDT=off
  PWM Generator4 : RelationalOperator  Operator=<=  OutDataTypeStr=boolean  InputSameDT=off
  Repeating Sequence1 : simulink/Sources/Repeating Sequence  rep_seq_t=[0, 1/2/fswitch, 1/fswitch ]  rep_seq_y=[0, 0.5, 1]
  Saturation{1..4} (4 alike) : Saturate  UpperLimit=1  LowerLimit=0
  Subtract : Sum  Inputs=-++
  Subtract1 : Sum
  Subtract2 : Sum  Inputs=-+
  PWM OUTPUT : Outport
  PWM OUTPUT N : Outport  Port=2
  Sample Trigger Output : Outport  Port=3
  wires:
  PWM CMP/1 -> Subtract2/1, Subtract1/1, Subtract/1, Data Type Conversion4/1
  Data Type Conversion4/1 -> Gain2/1
  Gain2/1 -> Saturation1/1
  Saturation1/1 -> PWM Generator1/1
  PWM Generator1/1 -> Logical Operator2/1
  Logical Operator2/1 -> Logical Operator3/2
  Constant1/1 -> Subtract/2
  Constant3/1 -> Subtract/3
  PWM Generator2/1 -> Logical Operator2/2
  Gain3/1 -> Saturation2/1
  Subtract/1 -> Gain3/1
  Saturation2/1 -> PWM Generator2/1
  Constant4/1 -> Subtract1/2
  Gain4/1 -> Saturation3/1
  Subtract1/1 -> Gain4/1
  Saturation3/1 -> PWM Generator3/2
  PWM Generator3/1 -> Logical Operator4/1
  Constant5/1 -> Subtract2/2
  Saturation4/1 -> PWM Generator4/2
  Gain5/1 -> Saturation4/1
  Subtract2/1 -> Gain5/1
  PWM Generator4/1 -> Logical Operator4/2
  Logical Operator4/1 -> Logical Operator5/2
  Repeating Sequence1/1 -> PWM Generator2/2, PWM Generator1/2, PWM Generator3/1, Hit Crossing：ADC Sample Trigger Signal/1, PWM Generator4/1
  Enable/1 -> Logical Operator5/1, Logical Operator3/1
  Logical Operator5/1 -> PWM OUTPUT N/1
  Logical Operator3/1 -> PWM OUTPUT/1
  Hit Crossing：ADC Sample Trigger Signal/1 -> Sample Trigger Output/1

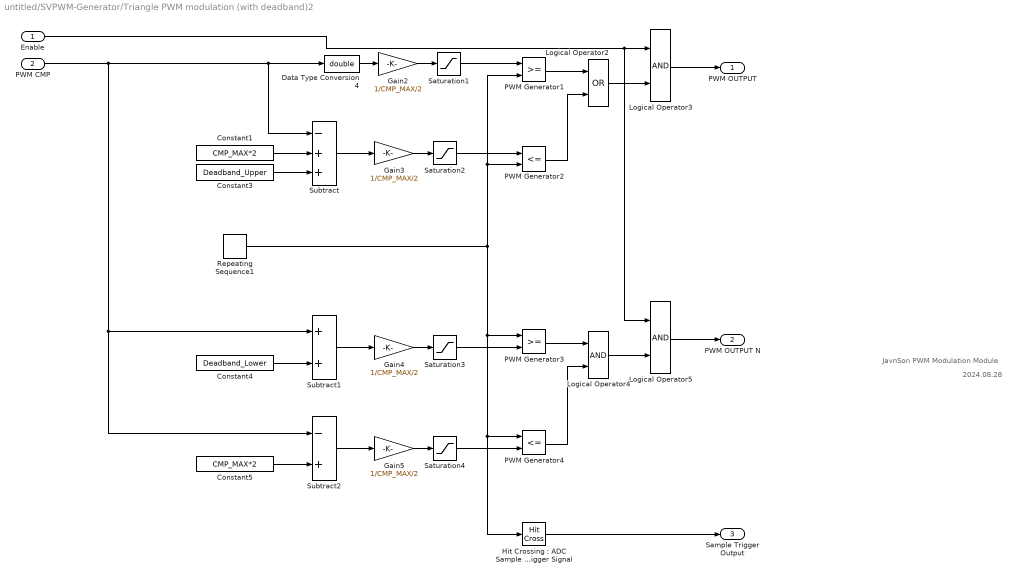
== system untitled/SVPWM-Generator/Triangle PWM modulation (with deadband)2 ==
  note: 2024.08.28
  note: JavnSon PWM Modulation Module
  Enable : Inport
  PWM CMP : Inport  Port=2
  Constant1 : Constant  Value=CMP_MAX*2
  Constant3 : Constant  Value=Deadband_Upper
  Constant4 : Constant  Value=Deadband_Lower
  Constant5 : Constant  Value=CMP_MAX*2
  Data Type Conversion4 : DataTypeConversion  OutDataTypeStr=double  SaturateOnIntegerOverflow=off  RndMeth=Floor
  Gain{2..5} (4 alike) : Gain  Gain=1/CMP_MAX/2
  Hit Crossing：ADC Sample Trigger Signal : HitCross  HitCrossingOffset=0.5  HitCrossingDirection=rising
  Logical Operator2 : Logic  Operator=OR  AllPortsSameDT=off  OutDataTypeStr=boolean
  Logical Operator3 : Logic  AllPortsSameDT=off  OutDataTypeStr=boolean
  Logical Operator4 : Logic  AllPortsSameDT=off  OutDataTypeStr=boolean
  Logical Operator5 : Logic  AllPortsSameDT=off  OutDataTypeStr=boolean
  PWM Generator1 : RelationalOperator  OutDataTypeStr=boolean  InputSameDT=off
  PWM Generator2 : RelationalOperator  Operator=<=  OutDataTypeStr=boolean  InputSameDT=off
  PWM Generator3 : RelationalOperator  OutDataTypeStr=boolean  InputSameDT=off
  PWM Generator4 : RelationalOperator  Operator=<=  OutDataTypeStr=boolean  InputSameDT=off
  Repeating Sequence1 : simulink/Sources/Repeating Sequence  rep_seq_t=[0, 1/2/fswitch, 1/fswitch ]  rep_seq_y=[0, 0.5, 1]
  Saturation{1..4} (4 alike) : Saturate  UpperLimit=1  LowerLimit=0
  Subtract : Sum  Inputs=-++
  Subtract1 : Sum
  Subtract2 : Sum  Inputs=-+
  PWM OUTPUT : Outport
  PWM OUTPUT N : Outport  Port=2
  Sample Trigger Output : Outport  Port=3
  wires:
  PWM CMP/1 -> Subtract2/1, Subtract1/1, Subtract/1, Data Type Conversion4/1
  Data Type Conversion4/1 -> Gain2/1
  Gain2/1 -> Saturation1/1
  Saturation1/1 -> PWM Generator1/1
  PWM Generator1/1 -> Logical Operator2/1
  Logical Operator2/1 -> Logical Operator3/2
  Constant1/1 -> Subtract/2
  Constant3/1 -> Subtract/3
  PWM Generator2/1 -> Logical Operator2/2
  Gain3/1 -> Saturation2/1
  Subtract/1 -> Gain3/1
  Saturation2/1 -> PWM Generator2/1
  Constant4/1 -> Subtract1/2
  Gain4/1 -> Saturation3/1
  Subtract1/1 -> Gain4/1
  Saturation3/1 -> PWM Generator3/2
  PWM Generator3/1 -> Logical Operator4/1
  Constant5/1 -> Subtract2/2
  Saturation4/1 -> PWM Generator4/2
  Gain5/1 -> Saturation4/1
  Subtract2/1 -> Gain5/1
  PWM Generator4/1 -> Logical Operator4/2
  Logical Operator4/1 -> Logical Operator5/2
  Repeating Sequence1/1 -> PWM Generator2/2, PWM Generator1/2, PWM Generator3/1, Hit Crossing：ADC Sample Trigger Signal/1, PWM Generator4/1
  Enable/1 -> Logical Operator5/1, Logical Operator3/1
  Logical Operator5/1 -> PWM OUTPUT N/1
  Logical Operator3/1 -> PWM OUTPUT/1
  Hit Crossing：ADC Sample Trigger Signal/1 -> Sample Trigger Output/1

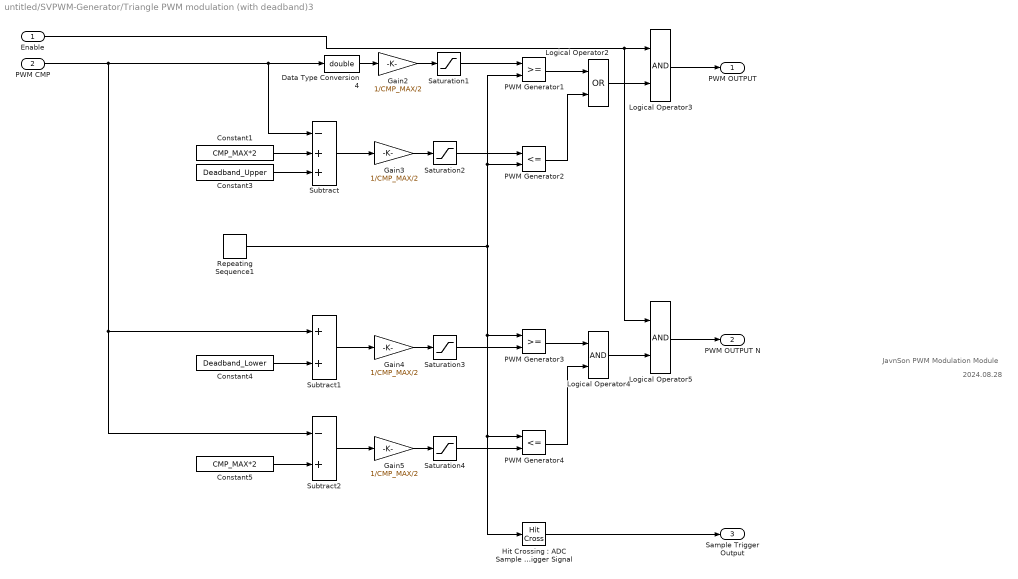
== system untitled/SVPWM-Generator/Triangle PWM modulation (with deadband)3 ==
  note: 2024.08.28
  note: JavnSon PWM Modulation Module
  Enable : Inport
  PWM CMP : Inport  Port=2
  Constant1 : Constant  Value=CMP_MAX*2
  Constant3 : Constant  Value=Deadband_Upper
  Constant4 : Constant  Value=Deadband_Lower
  Constant5 : Constant  Value=CMP_MAX*2
  Data Type Conversion4 : DataTypeConversion  OutDataTypeStr=double  SaturateOnIntegerOverflow=off  RndMeth=Floor
  Gain{2..5} (4 alike) : Gain  Gain=1/CMP_MAX/2
  Hit Crossing：ADC Sample Trigger Signal : HitCross  HitCrossingOffset=0.5  HitCrossingDirection=rising
  Logical Operator2 : Logic  Operator=OR  AllPortsSameDT=off  OutDataTypeStr=boolean
  Logical Operator3 : Logic  AllPortsSameDT=off  OutDataTypeStr=boolean
  Logical Operator4 : Logic  AllPortsSameDT=off  OutDataTypeStr=boolean
  Logical Operator5 : Logic  AllPortsSameDT=off  OutDataTypeStr=boolean
  PWM Generator1 : RelationalOperator  OutDataTypeStr=boolean  InputSameDT=off
  PWM Generator2 : RelationalOperator  Operator=<=  OutDataTypeStr=boolean  InputSameDT=off
  PWM Generator3 : RelationalOperator  OutDataTypeStr=boolean  InputSameDT=off
  PWM Generator4 : RelationalOperator  Operator=<=  OutDataTypeStr=boolean  InputSameDT=off
  Repeating Sequence1 : simulink/Sources/Repeating Sequence  rep_seq_t=[0, 1/2/fswitch, 1/fswitch ]  rep_seq_y=[0, 0.5, 1]
  Saturation{1..4} (4 alike) : Saturate  UpperLimit=1  LowerLimit=0
  Subtract : Sum  Inputs=-++
  Subtract1 : Sum
  Subtract2 : Sum  Inputs=-+
  PWM OUTPUT : Outport
  PWM OUTPUT N : Outport  Port=2
  Sample Trigger Output : Outport  Port=3
  wires:
  PWM CMP/1 -> Subtract2/1, Subtract1/1, Subtract/1, Data Type Conversion4/1
  Data Type Conversion4/1 -> Gain2/1
  Gain2/1 -> Saturation1/1
  Saturation1/1 -> PWM Generator1/1
  PWM Generator1/1 -> Logical Operator2/1
  Logical Operator2/1 -> Logical Operator3/2
  Constant1/1 -> Subtract/2
  Constant3/1 -> Subtract/3
  PWM Generator2/1 -> Logical Operator2/2
  Gain3/1 -> Saturation2/1
  Subtract/1 -> Gain3/1
  Saturation2/1 -> PWM Generator2/1
  Constant4/1 -> Subtract1/2
  Gain4/1 -> Saturation3/1
  Subtract1/1 -> Gain4/1
  Saturation3/1 -> PWM Generator3/2
  PWM Generator3/1 -> Logical Operator4/1
  Constant5/1 -> Subtract2/2
  Saturation4/1 -> PWM Generator4/2
  Gain5/1 -> Saturation4/1
  Subtract2/1 -> Gain5/1
  PWM Generator4/1 -> Logical Operator4/2
  Logical Operator4/1 -> Logical Operator5/2
  Repeating Sequence1/1 -> PWM Generator2/2, PWM Generator1/2, PWM Generator3/1, Hit Crossing：ADC Sample Trigger Signal/1, PWM Generator4/1
  Enable/1 -> Logical Operator5/1, Logical Operator3/1
  Logical Operator5/1 -> PWM OUTPUT N/1
  Logical Operator3/1 -> PWM OUTPUT/1
  Hit Crossing：ADC Sample Trigger Signal/1 -> Sample Trigger Output/1

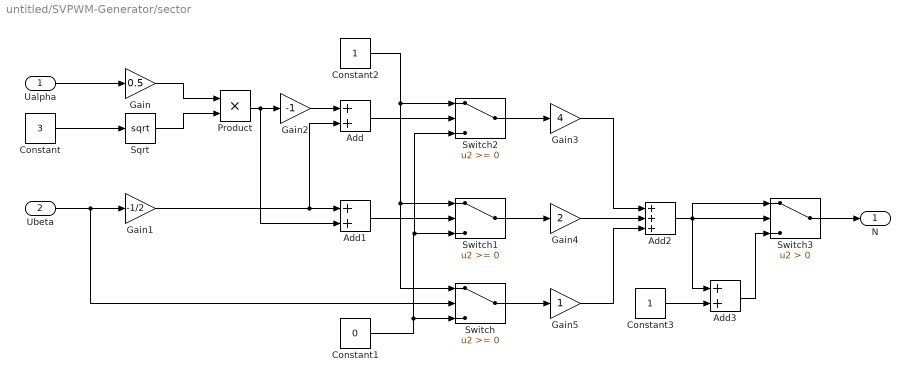
== system untitled/SVPWM-Generator/sector ==
  Ualpha : Inport
  Ubeta : Inport  Port=2
  Add : Sum
  Add1 : Sum
  Add2 : Sum  Inputs=+++
  Add3 : Sum
  Constant : Constant  Value=3
  Constant1 : Constant  Value=0
  Constant2 : Constant
  Constant3 : Constant
  Gain : Gain  Gain=0.5
  Gain1 : Gain  Gain=-1/2
  Gain2 : Gain  Gain=-1
  Gain3 : Gain  Gain=4
  Gain4 : Gain  Gain=2
  Gain5 : Gain
  Product : Product
  Sqrt : Sqrt
  Switch : Switch  SaturateOnIntegerOverflow=off  InputSameDT=off
  Switch1 : Switch  SaturateOnIntegerOverflow=off  InputSameDT=off
  Switch2 : Switch  SaturateOnIntegerOverflow=off  InputSameDT=off
  Switch3 : Switch  Criteria=u2 > Threshold  SaturateOnIntegerOverflow=off  InputSameDT=off
  N : Outport
  wires:
  Gain1/1 -> Add1/1, Add/2
  Constant1/1 -> Switch2/3, Switch1/3, Switch/3
  Gain2/1 -> Add/1
  Gain/1 -> Product/1
  Constant3/1 -> Add3/2
  Add/1 -> Switch2/2
  Product/1 -> Add1/2, Gain2/1
  Sqrt/1 -> Product/2
  Ubeta/1 -> Switch/2, Gain1/1
  Switch/1 -> Gain5/1
  Switch2/1 -> Gain3/1
  Add3/1 -> Switch3/3
  Add2/1 -> Switch3/1, Add3/1, Switch3/2
  Switch3/1 -> N/1
  Gain3/1 -> Add2/1
  Add1/1 -> Switch1/2
  Switch1/1 -> Gain4/1
  Gain4/1 -> Add2/2
  Constant/1 -> Sqrt/1
  Gain5/1 -> Add2/3
  Constant2/1 -> Switch/1, Switch1/1, Switch2/1
  Ualpha/1 -> Gain/1

== system untitled/Three Phase Driver Model/Single Phase Full Bridge ==
  Enable : Inport
  PWM CMP : Inport  Port=2
  Mosfet8 : spsMosfetLib/Mosfet  Ron=0.1  Lon=0  Rd=0.01  Vfd=0  IC=0  Rs=1e5  Cs=inf  Measurements=off
  Mosfet9 : spsMosfetLib/Mosfet  Ron=0.1  Lon=0  Rd=0.01  Vfd=0  IC=0  Rs=1e5  Cs=inf  Measurements=off
  Triangle PWM modulation (with deadband)3 : Subsystem  mask{fswitch=10e3, CMP_MAX=10000, Deadband_Upper=0, Deadband_Lower=0, Parameter4=0}
      mask prompts: Parameter4 "Deadband Time: (μs)"
      mask Callback Deadband_Upper: %dead_cmp_param = get_param('DEADBAND_CMP','Value');
      mask DialogControl DescGroupVar Prompt: PWM Modulator
      mask DialogControl DescTextVar Prompt: PWM Modulator. Input PWM compare register value, output ADC trigger signal, PWM output and negtive PWM output.
      mask DialogControl ParameterGroupVar Prompt: 参数
      mask DialogControl Control2 Prompt: PWM Frequency (Hz) :
      mask DialogControl Control4 Prompt: Full Scale PWM Compare value:
      mask DialogControl Control5 Prompt: (whole period is 2 * CMP_MAX ticks)
      mask DialogControl Control3 Prompt: Deadband Range Set (CMP Value):
      mask DialogControl Control6 Prompt: Single side deadband time: DEADBAND_CMP/2/CMP_MAX/fswitch
  D : PMIOPort  Side=Left
  Phase : PMIOPort  Port=2  Side=Right
  S : PMIOPort  Port=3  Side=Right
  Sample Trigger Output : Outport
  wires:
  Triangle PWM modulation (with deadband)3/1(PWM OUTPUT) -> Mosfet8/1
  Enable/1 -> Triangle PWM modulation (with deadband)3/1(Enable)
  Triangle PWM modulation (with deadband)3/3(Sample Trigger Output) -> Sample Trigger Output/1
  Triangle PWM modulation (with deadband)3/2(PWM OUTPUT N) -> Mosfet9/1
  PWM CMP/1 -> Triangle PWM modulation (with deadband)3/2(PWM CMP)
  connections:
  Mosfet8/LConn1 -- D/RConn1
  Mosfet9/LConn1 -- Phase/RConn1 -- Mosfet8/RConn1
  Mosfet9/RConn1 -- S/RConn1

== system untitled/Three Phase Driver Model/Single Phase Full Bridge1 ==
  Enable : Inport
  PWM CMP : Inport  Port=2
  Mosfet8 : spsMosfetLib/Mosfet  Ron=0.1  Lon=0  Rd=0.01  Vfd=0  IC=0  Rs=1e5  Cs=inf  Measurements=off
  Mosfet9 : spsMosfetLib/Mosfet  Ron=0.1  Lon=0  Rd=0.01  Vfd=0  IC=0  Rs=1e5  Cs=inf  Measurements=off
  Triangle PWM modulation (with deadband)3 : Subsystem  mask{fswitch=10e3, CMP_MAX=10000, Deadband_Upper=0, Deadband_Lower=0, Parameter4=0}
      mask prompts: Parameter4 "Deadband Time: (μs)"
      mask Callback Deadband_Upper: %dead_cmp_param = get_param('DEADBAND_CMP','Value');
      mask DialogControl DescGroupVar Prompt: PWM Modulator
      mask DialogControl DescTextVar Prompt: PWM Modulator. Input PWM compare register value, output ADC trigger signal, PWM output and negtive PWM output.
      mask DialogControl ParameterGroupVar Prompt: 参数
      mask DialogControl Control2 Prompt: PWM Frequency (Hz) :
      mask DialogControl Control4 Prompt: Full Scale PWM Compare value:
      mask DialogControl Control5 Prompt: (whole period is 2 * CMP_MAX ticks)
      mask DialogControl Control3 Prompt: Deadband Range Set (CMP Value):
      mask DialogControl Control6 Prompt: Single side deadband time: DEADBAND_CMP/2/CMP_MAX/fswitch
  D : PMIOPort  Side=Left
  Phase : PMIOPort  Port=2  Side=Right
  S : PMIOPort  Port=3  Side=Right
  Sample Trigger Output : Outport
  wires:
  Triangle PWM modulation (with deadband)3/1(PWM OUTPUT) -> Mosfet8/1
  Enable/1 -> Triangle PWM modulation (with deadband)3/1(Enable)
  Triangle PWM modulation (with deadband)3/3(Sample Trigger Output) -> Sample Trigger Output/1
  Triangle PWM modulation (with deadband)3/2(PWM OUTPUT N) -> Mosfet9/1
  PWM CMP/1 -> Triangle PWM modulation (with deadband)3/2(PWM CMP)
  connections:
  Mosfet8/LConn1 -- D/RConn1
  Mosfet8/RConn1 -- Mosfet9/LConn1 -- Phase/RConn1
  Mosfet9/RConn1 -- S/RConn1

== system untitled/Three Phase Driver Model/Single Phase Full Bridge2 ==
  Enable : Inport
  PWM CMP : Inport  Port=2
  Mosfet8 : spsMosfetLib/Mosfet  Ron=0.1  Lon=0  Rd=0.01  Vfd=0  IC=0  Rs=1e5  Cs=inf  Measurements=off
  Mosfet9 : spsMosfetLib/Mosfet  Ron=0.1  Lon=0  Rd=0.01  Vfd=0  IC=0  Rs=1e5  Cs=inf  Measurements=off
  Triangle PWM modulation (with deadband)3 : Subsystem  mask{fswitch=10e3, CMP_MAX=10000, Deadband_Upper=0, Deadband_Lower=0, Parameter4=0}
      mask prompts: Parameter4 "Deadband Time: (μs)"
      mask Callback Deadband_Upper: %dead_cmp_param = get_param('DEADBAND_CMP','Value');
      mask DialogControl DescGroupVar Prompt: PWM Modulator
      mask DialogControl DescTextVar Prompt: PWM Modulator. Input PWM compare register value, output ADC trigger signal, PWM output and negtive PWM output.
      mask DialogControl ParameterGroupVar Prompt: 参数
      mask DialogControl Control2 Prompt: PWM Frequency (Hz) :
      mask DialogControl Control4 Prompt: Full Scale PWM Compare value:
      mask DialogControl Control5 Prompt: (whole period is 2 * CMP_MAX ticks)
      mask DialogControl Control3 Prompt: Deadband Range Set (CMP Value):
      mask DialogControl Control6 Prompt: Single side deadband time: DEADBAND_CMP/2/CMP_MAX/fswitch
  D : PMIOPort  Side=Left
  Phase : PMIOPort  Port=2  Side=Right
  S : PMIOPort  Port=3  Side=Right
  Sample Trigger Output : Outport
  wires:
  Triangle PWM modulation (with deadband)3/1(PWM OUTPUT) -> Mosfet8/1
  Enable/1 -> Triangle PWM modulation (with deadband)3/1(Enable)
  Triangle PWM modulation (with deadband)3/3(Sample Trigger Output) -> Sample Trigger Output/1
  Triangle PWM modulation (with deadband)3/2(PWM OUTPUT N) -> Mosfet9/1
  PWM CMP/1 -> Triangle PWM modulation (with deadband)3/2(PWM CMP)
  connections:
  Mosfet8/LConn1 -- D/RConn1
  Mosfet8/RConn1 -- Mosfet9/LConn1 -- Phase/RConn1
  Mosfet9/RConn1 -- S/RConn1

== system untitled/Three Phase Driver Model1/Single Phase Full Bridge ==
  Enable : Inport
  PWM CMP : Inport  Port=2
  Mosfet8 : spsMosfetLib/Mosfet  Ron=1e-3  Lon=0  Rd=0.01  Vfd=0  IC=0  Rs=1e5  Cs=inf  Measurements=off
  Mosfet9 : spsMosfetLib/Mosfet  Ron=1e-3  Lon=0  Rd=0.01  Vfd=0  IC=0  Rs=1e5  Cs=inf  Measurements=off
  Triangle PWM modulation (with deadband)3 : Subsystem  mask{fswitch=10e3, CMP_MAX=10000, Deadband_Upper=0, Deadband_Lower=0, Parameter4=0}
      mask prompts: Parameter4 "Deadband Time: (μs)"
      mask Callback Deadband_Upper: %dead_cmp_param = get_param('DEADBAND_CMP','Value');
      mask DialogControl DescGroupVar Prompt: PWM Modulator
      mask DialogControl DescTextVar Prompt: PWM Modulator. Input PWM compare register value, output ADC trigger signal, PWM output and negtive PWM output.
      mask DialogControl ParameterGroupVar Prompt: 参数
      mask DialogControl Control2 Prompt: PWM Frequency (Hz) :
      mask DialogControl Control4 Prompt: Full Scale PWM Compare value:
      mask DialogControl Control5 Prompt: (whole period is 2 * CMP_MAX ticks)
      mask DialogControl Control3 Prompt: Deadband Range Set (CMP Value):
      mask DialogControl Control6 Prompt: Single side deadband time: DEADBAND_CMP/2/CMP_MAX/fswitch
  D : PMIOPort  Side=Left
  Phase : PMIOPort  Port=2  Side=Right
  S : PMIOPort  Port=3  Side=Right
  Sample Trigger Output : Outport
  wires:
  Triangle PWM modulation (with deadband)3/1(PWM OUTPUT) -> Mosfet8/1
  Enable/1 -> Triangle PWM modulation (with deadband)3/1(Enable)
  Triangle PWM modulation (with deadband)3/3(Sample Trigger Output) -> Sample Trigger Output/1
  Triangle PWM modulation (with deadband)3/2(PWM OUTPUT N) -> Mosfet9/1
  PWM CMP/1 -> Triangle PWM modulation (with deadband)3/2(PWM CMP)
  connections:
  Mosfet8/LConn1 -- D/RConn1
  Mosfet9/LConn1 -- Phase/RConn1 -- Mosfet8/RConn1
  Mosfet9/RConn1 -- S/RConn1

== system untitled/Three Phase Driver Model1/Single Phase Full Bridge1 ==
  Enable : Inport
  PWM CMP : Inport  Port=2
  Mosfet8 : spsMosfetLib/Mosfet  Ron=1e-3  Lon=0  Rd=0.01  Vfd=0  IC=0  Rs=1e5  Cs=inf  Measurements=off
  Mosfet9 : spsMosfetLib/Mosfet  Ron=1e-3  Lon=0  Rd=0.01  Vfd=0  IC=0  Rs=1e5  Cs=inf  Measurements=off
  Triangle PWM modulation (with deadband)3 : Subsystem  mask{fswitch=10e3, CMP_MAX=10000, Deadband_Upper=0, Deadband_Lower=0, Parameter4=0}
      mask prompts: Parameter4 "Deadband Time: (μs)"
      mask Callback Deadband_Upper: %dead_cmp_param = get_param('DEADBAND_CMP','Value');
      mask DialogControl DescGroupVar Prompt: PWM Modulator
      mask DialogControl DescTextVar Prompt: PWM Modulator. Input PWM compare register value, output ADC trigger signal, PWM output and negtive PWM output.
      mask DialogControl ParameterGroupVar Prompt: 参数
      mask DialogControl Control2 Prompt: PWM Frequency (Hz) :
      mask DialogControl Control4 Prompt: Full Scale PWM Compare value:
      mask DialogControl Control5 Prompt: (whole period is 2 * CMP_MAX ticks)
      mask DialogControl Control3 Prompt: Deadband Range Set (CMP Value):
      mask DialogControl Control6 Prompt: Single side deadband time: DEADBAND_CMP/2/CMP_MAX/fswitch
  D : PMIOPort  Side=Left
  Phase : PMIOPort  Port=2  Side=Right
  S : PMIOPort  Port=3  Side=Right
  Sample Trigger Output : Outport
  wires:
  Triangle PWM modulation (with deadband)3/1(PWM OUTPUT) -> Mosfet8/1
  Enable/1 -> Triangle PWM modulation (with deadband)3/1(Enable)
  Triangle PWM modulation (with deadband)3/3(Sample Trigger Output) -> Sample Trigger Output/1
  Triangle PWM modulation (with deadband)3/2(PWM OUTPUT N) -> Mosfet9/1
  PWM CMP/1 -> Triangle PWM modulation (with deadband)3/2(PWM CMP)
  connections:
  Mosfet8/LConn1 -- D/RConn1
  Mosfet8/RConn1 -- Mosfet9/LConn1 -- Phase/RConn1
  Mosfet9/RConn1 -- S/RConn1

== system untitled/Three Phase Driver Model1/Single Phase Full Bridge2 ==
  Enable : Inport
  PWM CMP : Inport  Port=2
  Mosfet8 : spsMosfetLib/Mosfet  Ron=1e-3  Lon=0  Rd=0.01  Vfd=0  IC=0  Rs=1e5  Cs=inf  Measurements=off
  Mosfet9 : spsMosfetLib/Mosfet  Ron=1e-3  Lon=0  Rd=0.01  Vfd=0  IC=0  Rs=1e5  Cs=inf  Measurements=off
  Triangle PWM modulation (with deadband)3 : Subsystem  mask{fswitch=10e3, CMP_MAX=10000, Deadband_Upper=0, Deadband_Lower=0, Parameter4=0}
      mask prompts: Parameter4 "Deadband Time: (μs)"
      mask Callback Deadband_Upper: %dead_cmp_param = get_param('DEADBAND_CMP','Value');
      mask DialogControl DescGroupVar Prompt: PWM Modulator
      mask DialogControl DescTextVar Prompt: PWM Modulator. Input PWM compare register value, output ADC trigger signal, PWM output and negtive PWM output.
      mask DialogControl ParameterGroupVar Prompt: 参数
      mask DialogControl Control2 Prompt: PWM Frequency (Hz) :
      mask DialogControl Control4 Prompt: Full Scale PWM Compare value:
      mask DialogControl Control5 Prompt: (whole period is 2 * CMP_MAX ticks)
      mask DialogControl Control3 Prompt: Deadband Range Set (CMP Value):
      mask DialogControl Control6 Prompt: Single side deadband time: DEADBAND_CMP/2/CMP_MAX/fswitch
  D : PMIOPort  Side=Left
  Phase : PMIOPort  Port=2  Side=Right
  S : PMIOPort  Port=3  Side=Right
  Sample Trigger Output : Outport
  wires:
  Triangle PWM modulation (with deadband)3/1(PWM OUTPUT) -> Mosfet8/1
  Enable/1 -> Triangle PWM modulation (with deadband)3/1(Enable)
  Triangle PWM modulation (with deadband)3/3(Sample Trigger Output) -> Sample Trigger Output/1
  Triangle PWM modulation (with deadband)3/2(PWM OUTPUT N) -> Mosfet9/1
  PWM CMP/1 -> Triangle PWM modulation (with deadband)3/2(PWM CMP)
  connections:
  Mosfet8/LConn1 -- D/RConn1
  Mosfet8/RConn1 -- Mosfet9/LConn1 -- Phase/RConn1
  Mosfet9/RConn1 -- S/RConn1
